simulink model "threePhase_SVPWM"  (R2022b)
settings: Solver=FixedStepAuto  StartTime=0.0  StopTime=0.02  RelTol=1e-3  EnableMultiTasking=on
values from neighbouring files (symbols this model uses):
  Vs = 230    [QuartusPath.m]
undefined symbols (not defined in the file or in its folder): Add, Shift
libraries: simulink x19, dspsrcs4 x3, dsphdlmathfun2 x1
settings Model: Creator=BAYINDIR  LastModifiedBy=BAYINDIR
settings OptimizationCC: BlockReduction=off  ConditionallyExecuteInputs=off
settings DebuggingCC: SingleTaskRateTransMsg=error

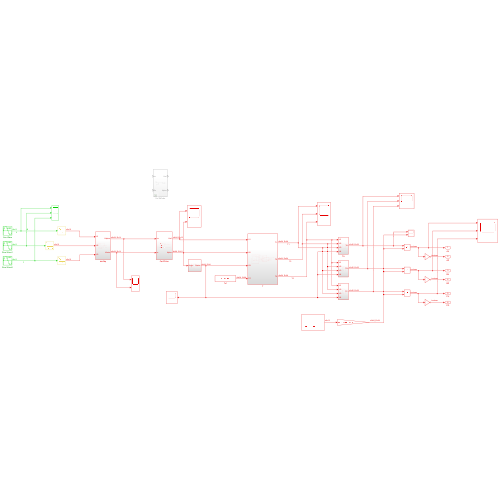
[thumbnail: Simulink's stored preview of the top-level diagram]
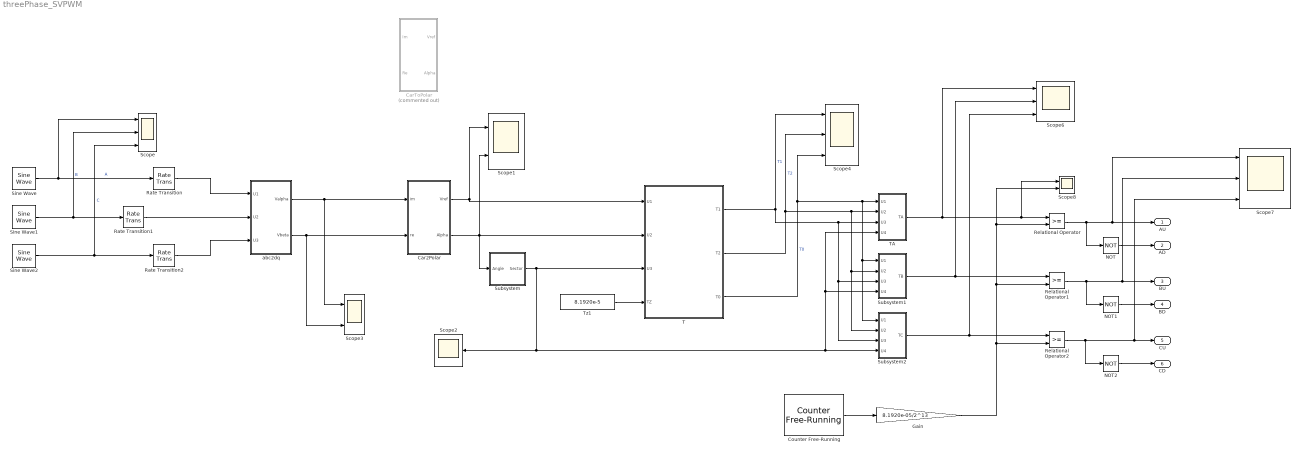
== system threePhase_SVPWM ==
  Car2Polar : Subsystem
  CarToPolar : Subsystem  Commented=on
  Counter Free-Running : simulink/Sources/Counter Free-Running  NumBits=13  tsamp=-1
  Gain : Gain  Gain=8.1920e-05/2^13  ParamDataTypeStr=fixdt(0,32,32)  OutDataTypeStr=fixdt(0,24,24)
  NOT : Logic  Operator=NOT  IconShape=distinctive  AllPortsSameDT=off  OutDataTypeStr=boolean
  NOT1 : Logic  Operator=NOT  IconShape=distinctive  AllPortsSameDT=off  OutDataTypeStr=boolean
  NOT2 : Logic  Operator=NOT  IconShape=distinctive  AllPortsSameDT=off  OutDataTypeStr=boolean
  Rate Transition : RateTransition  OutPortSampleTime=1/100000000
  Rate Transition1 : RateTransition  OutPortSampleTime=1/100000000
  Rate Transition2 : RateTransition  OutPortSampleTime=1/100000000
  Relational Operator : RelationalOperator  OutDataTypeStr=boolean  RndMeth=Simplest  InputSameDT=off
  Relational Operator1 : RelationalOperator  OutDataTypeStr=boolean  RndMeth=Simplest  InputSameDT=off
  Relational Operator2 : RelationalOperator  OutDataTypeStr=boolean  RndMeth=Simplest  InputSameDT=off
  Scope{,4,6..7} (4 alike) : Scope  NumInputPorts=3
  Scope1 : Scope  NumInputPorts=2
  Scope2 : Scope
  Scope3 : Scope  NumInputPorts=2
  Scope8 : Scope  NumInputPorts=2
  Sine Wave : dspsrcs4/Sine Wave  Amplitude=Vs  Frequency=50  Phase=0  SampleMode=Discrete  OutComplex=Real  CompMethod=Table lookup  TableSize=Speed  SampleTime=1/1000000  SamplesPerFrame=1  ResetState=Restart at time zero  OutputFrames=off  dataType=Fixed-point  wordLen=12  udDataType=sfix(16)  fracBitsMode=User-defined  numFracBits=0  OutDataTypeStr=fixdt(1,12,0)  LastOutDataTypeStr=fixdt(1,12,0)
  Sine Wave1 : dspsrcs4/Sine Wave  Amplitude=Vs  Frequency=50  Phase=2*pi/3  SampleMode=Discrete  OutComplex=Real  CompMethod=Table lookup  TableSize=Speed  SampleTime=1/1000000  SamplesPerFrame=1  ResetState=Restart at time zero  OutputFrames=off  dataType=Fixed-point  wordLen=12  udDataType=sfix(16)  fracBitsMode=User-defined  numFracBits=0  OutDataTypeStr=fixdt(1,12,0)  LastOutDataTypeStr=fixdt(1,12,0)
  Sine Wave2 : dspsrcs4/Sine Wave  Amplitude=Vs  Frequency=50  Phase=4*pi/3  SampleMode=Discrete  OutComplex=Real  CompMethod=Table lookup  TableSize=Speed  SampleTime=1/1000000  SamplesPerFrame=1  ResetState=Restart at time zero  OutputFrames=off  dataType=Fixed-point  wordLen=12  udDataType=sfix(16)  fracBitsMode=User-defined  numFracBits=0  OutDataTypeStr=fixdt(1,12,0)  LastOutDataTypeStr=fixdt(1,12,0)
  Subsystem : Subsystem
  Subsystem1 : Subsystem
  Subsystem2 : Subsystem
  T : Subsystem
  TA : Subsystem
  Tz1 : Constant  Value=8.1920e-5  OutDataTypeStr=fixdt(0,24,24)  SampleTime=-1
  abc2dq : Subsystem
  AU : Outport
  AD : Outport  Port=2
  BU : Outport  Port=3
  BD : Outport  Port=4
  CU : Outport  Port=5
  CD : Outport  Port=6
  wires:
  Sine Wave/1 -> Rate Transition/1, Scope/1  "A"
  Sine Wave1/1 -> Rate Transition1/1, Scope/2  "B"
  Sine Wave2/1 -> Rate Transition2/1, Scope/3  "C"
  Rate Transition/1 -> abc2dq/1(U1)
  Rate Transition1/1 -> abc2dq/2(U2)
  Rate Transition2/1 -> abc2dq/3(U3)
  Car2Polar/1(Vref) -> Scope1/1, T/1(U1)
  Car2Polar/2(Alpha) -> Scope1/2, Subsystem/1(Angle), T/2(U2)
  Subsystem/1(Sector) -> T/3(U3), TA/4(U4), Subsystem1/4(U4), Subsystem2/4(U4), Scope2/1
  Tz1/1 -> T/4(TZ)
  T/1(T1) -> TA/3(U3), Subsystem2/3(U3), Subsystem1/3(U3), Scope4/1  "T1"
  T/2(T2) -> Scope4/2, Subsystem1/2(U2), Subsystem2/2(U2), TA/2(U2)  "T2"
  T/3(T0) -> Scope4/3, Subsystem2/1(U1), Subsystem1/1(U1), TA/1(U1)  "T0"
  TA/1(TA) -> Scope8/1, Relational Operator/1, Scope6/1
  abc2dq/2(Vbeta) -> Car2Polar/2(re), Scope3/2
  abc2dq/1(Valpha) -> Scope3/1, Car2Polar/1(im)
  Subsystem1/1(TB) -> Relational Operator1/1, Scope6/2
  Subsystem2/1(TC) -> Relational Operator2/1, Scope6/3
  Counter Free-Running/1 -> Gain/1
  Relational Operator/1 -> NOT/1, Scope7/1, AU/1
  NOT/1 -> AD/1
  NOT1/1 -> BD/1
  Relational Operator1/1 -> NOT1/1, Scope7/2, BU/1
  Relational Operator2/1 -> Scope7/3, CU/1, NOT2/1
  NOT2/1 -> CD/1
  Gain/1 -> Scope8/2, Relational Operator/2, Relational Operator1/2, Relational Operator2/2

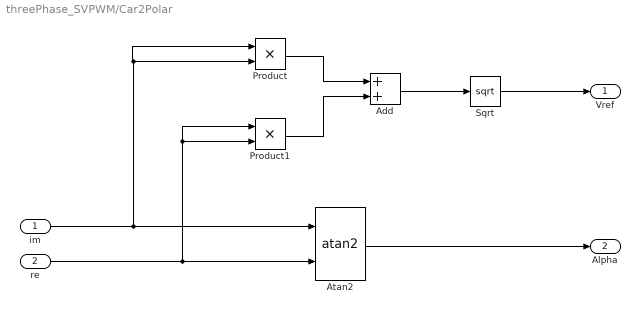
== system threePhase_SVPWM/Car2Polar ==
  im : Inport
  re : Inport  Port=2
  Add : Sum  OutDataTypeStr=fixdt(0,24,8)
  Atan2 : Trigonometry  Operator=atan2  ApproximationMethod=CORDIC  NumberOfIterations=13
  Product : Product  OutDataTypeStr=fixdt(1,48,28)
  Product1 : Product  OutDataTypeStr=fixdt(1,48,28)
  Sqrt : Sqrt  OutDataTypeStr=fixdt(0,24,12)
  Vref : Outport
  Alpha : Outport  Port=2
  wires:
  re/1 -> Product1/2, Product1/1, Atan2/2
  Atan2/1 -> Alpha/1
  im/1 -> Product/2, Product/1, Atan2/1
  Product/1 -> Add/1
  Product1/1 -> Add/2
  Add/1 -> Sqrt/1
  Sqrt/1 -> Vref/1

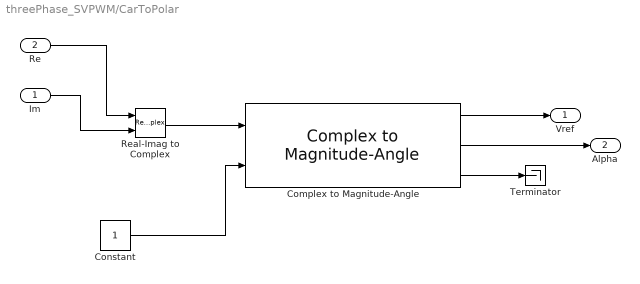
== system threePhase_SVPWM/CarToPolar ==
  Im : Inport
  Re : Inport  Port=2
  Complex to Magnitude-Angle : dsphdlmathfun2/Complex to Magnitude-Angle  NumIterationsSource=Property  NumIterations=12  OutputFormat=Magnitude and angle  AngleFormat=Radians  ScaleOutput=on  ScalingMethod=Shift-Add  SimulateUsing=Code generation
  Constant : Constant  OutDataTypeStr=boolean  SampleTime=-1
  Real-Imag to Complex : RealImagToComplex
  Terminator : Terminator
  Vref : Outport
  Alpha : Outport  Port=2
  wires:
  Im/1 -> Real-Imag to Complex/2
  Real-Imag to Complex/1 -> Complex to Magnitude-Angle/1
  Complex to Magnitude-Angle/3 -> Terminator/1
  Complex to Magnitude-Angle/2 -> Alpha/1
  Re/1 -> Real-Imag to Complex/1
  Constant/1 -> Complex to Magnitude-Angle/2
  Complex to Magnitude-Angle/1 -> Vref/1

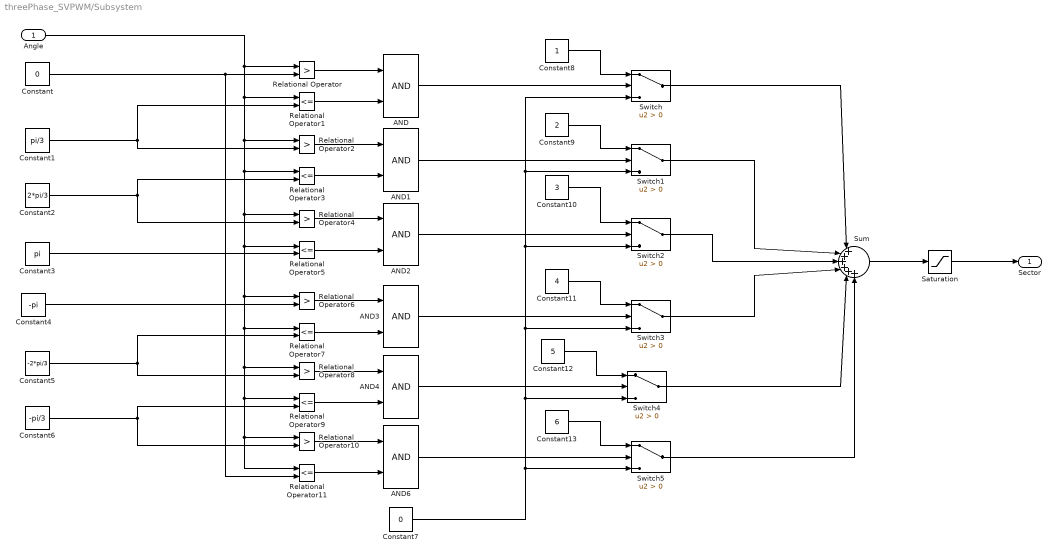
== system threePhase_SVPWM/Subsystem ==
  Angle : Inport
  AND{,1..4,6} (6 alike) : Logic  IconShape=distinctive  AllPortsSameDT=off  OutDataTypeStr=boolean
  Constant : Constant  Value=0  OutDataTypeStr=fixdt(1,27,24)  SampleTime=-1
  Constant1 : Constant  Value=pi/3  OutDataTypeStr=fixdt(1,27,24)  SampleTime=-1
  Constant10 : Constant  Value=3  OutDataTypeStr=fixdt(1,16,8)  SampleTime=-1
  Constant11 : Constant  Value=4  OutDataTypeStr=fixdt(1,16,8)  SampleTime=-1
  Constant12 : Constant  Value=5  OutDataTypeStr=fixdt(1,16,8)  SampleTime=-1
  Constant13 : Constant  Value=6  OutDataTypeStr=fixdt(1,16,8)  SampleTime=-1
  Constant2 : Constant  Value=2*pi/3  OutDataTypeStr=fixdt(1,27,24)  SampleTime=-1
  Constant3 : Constant  Value=pi  OutDataTypeStr=fixdt(1,27,24)  SampleTime=-1
  Constant4 : Constant  Value=-pi  OutDataTypeStr=fixdt(1,27,24)  SampleTime=-1
  Constant5 : Constant  Value=-2*pi/3  OutDataTypeStr=fixdt(1,27,24)  SampleTime=-1
  Constant6 : Constant  Value=-pi/3  OutDataTypeStr=fixdt(1,27,24)  SampleTime=-1
  Constant7 : Constant  Value=0  OutDataTypeStr=fixdt(1,16,8)  SampleTime=-1
  Constant8 : Constant  OutDataTypeStr=fixdt(1,16,8)  SampleTime=-1
  Constant9 : Constant  Value=2  OutDataTypeStr=fixdt(1,16,8)  SampleTime=-1
  Relational Operator{,2,4,6,8,10} (6 alike) : RelationalOperator  Operator=>  OutDataTypeStr=boolean  RndMeth=Simplest  InputSameDT=off
  Relational Operator{1,3,5,7,9,11} (6 alike) : RelationalOperator  Operator=<=  OutDataTypeStr=boolean  RndMeth=Simplest  InputSameDT=off
  Saturation : Saturate  UpperLimit=6  LowerLimit=1
  Sum : Sum  Inputs=|++++++  OutDataTypeStr=fixdt(0,16,8)
  Switch{,1..5} (6 alike) : Switch  Criteria=u2 > Threshold  SaturateOnIntegerOverflow=off  InputSameDT=off
  Sector : Outport
  wires:
  Angle/1 -> Relational Operator/1, Relational Operator10/1, Relational Operator11/1, Relational Operator9/1, Relational Operator8/1, Relational Operator7/1, Relational Operator6/1, Relational Operator5/1, Relational Operator4/1, Relational Operator3/1, Relational Operator2/1, Relational Operator1/1
  Relational Operator/1 -> AND/1
  AND4/1 -> Switch4/2
  Constant7/1 -> Switch5/3, Switch4/3, Switch3/3, Switch2/3, Switch1/3, Switch/3
  Saturation/1 -> Sector/1
  Constant9/1 -> Switch1/1
  Constant5/1 -> Relational Operator7/2, Relational Operator8/2
  Relational Operator6/1 -> AND3/1
  Constant1/1 -> Relational Operator2/2, Relational Operator1/2
  Switch1/1 -> Sum/2
  Relational Operator11/1 -> AND6/2
  Constant3/1 -> Relational Operator5/2
  Switch/1 -> Sum/1
  Sum/1 -> Saturation/1
  Constant10/1 -> Switch2/1
  Relational Operator5/1 -> AND2/2
  Constant13/1 -> Switch5/1
  Constant8/1 -> Switch/1
  Switch2/1 -> Sum/3
  AND1/1 -> Switch1/2
  AND6/1 -> Switch5/2
  Relational Operator10/1 -> AND6/1
  Switch5/1 -> Sum/6
  Constant2/1 -> Relational Operator4/2, Relational Operator3/2
  Relational Operator1/1 -> AND/2
  Constant4/1 -> Relational Operator6/2
  Relational Operator4/1 -> AND2/1
  Constant/1 -> Relational Operator11/2, Relational Operator/2
  Constant6/1 -> Relational Operator9/2, Relational Operator10/2
  Switch4/1 -> Sum/5
  Constant12/1 -> Switch4/1
  Constant11/1 -> Switch3/1
  Relational Operator7/1 -> AND3/2
  AND3/1 -> Switch3/2
  AND/1 -> Switch/2
  Switch3/1 -> Sum/4
  Relational Operator9/1 -> AND4/2
  Relational Operator3/1 -> AND1/2
  Relational Operator2/1 -> AND1/1
  AND2/1 -> Switch2/2
  Relational Operator8/1 -> AND4/1

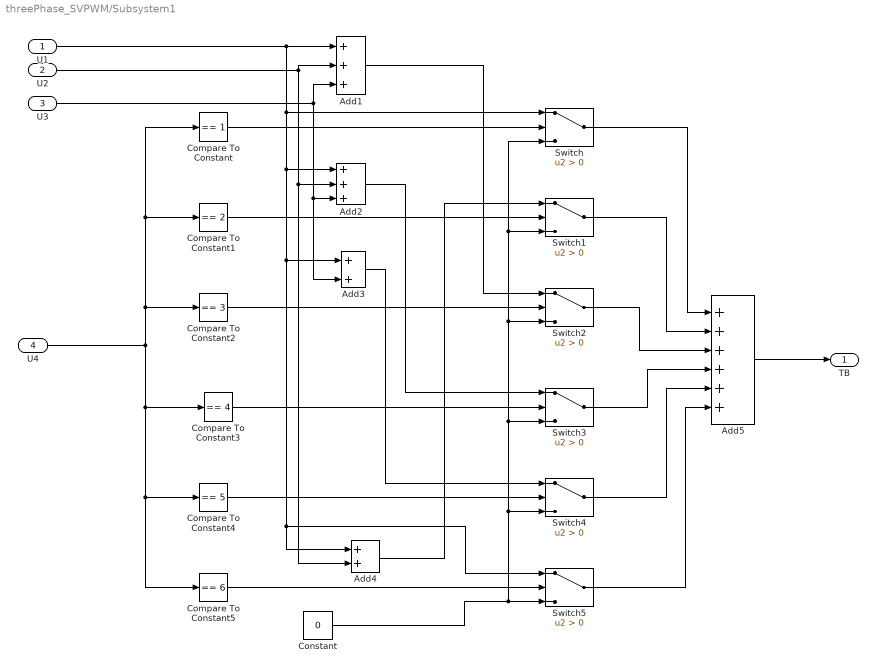
== system threePhase_SVPWM/Subsystem1 ==
  U1 : Inport
  U2 : Inport  Port=2
  U3 : Inport  Port=3
  U4 : Inport  Port=4
  Add1 : Sum  Inputs=+++  OutDataTypeStr=fixdt(0,24,24)
  Add2 : Sum  Inputs=+++  OutDataTypeStr=fixdt(0,24,24)
  Add3 : Sum  OutDataTypeStr=fixdt(0,24,24)
  Add4 : Sum  OutDataTypeStr=fixdt(0,24,24)
  Add5 : Sum  Inputs=++++++  OutDataTypeStr=fixdt(0,32,32)
  Compare To Constant : simulink/Logic and Bit Operations/Compare To Constant  relop===  const=1  OutDataTypeStr=boolean
  Compare To Constant1 : simulink/Logic and Bit Operations/Compare To Constant  relop===  const=2  OutDataTypeStr=boolean
  Compare To Constant2 : simulink/Logic and Bit Operations/Compare To Constant  relop===  const=3  OutDataTypeStr=boolean
  Compare To Constant3 : simulink/Logic and Bit Operations/Compare To Constant  relop===  const=4  OutDataTypeStr=boolean
  Compare To Constant4 : simulink/Logic and Bit Operations/Compare To Constant  relop===  const=5  OutDataTypeStr=boolean
  Compare To Constant5 : simulink/Logic and Bit Operations/Compare To Constant  relop===  const=6  OutDataTypeStr=boolean
  Constant : Constant  Value=0  OutDataTypeStr=uint8  SampleTime=-1
  Switch{,1..5} (6 alike) : Switch  Criteria=u2 > Threshold  OutDataTypeStr=fixdt(0,24,24)  SaturateOnIntegerOverflow=off  InputSameDT=off
  TB : Outport
  wires:
  U1/1 -> Switch5/1, Add4/1, Add3/1, Add2/1, Switch/1, Add1/1
  Compare To Constant4/1 -> Switch4/2
  Switch4/1 -> Add5/5
  Switch1/1 -> Add5/2
  U4/1 -> Compare To Constant2/1, Compare To Constant1/1, Compare To Constant/1, Compare To Constant4/1, Compare To Constant5/1, Compare To Constant3/1
  Compare To Constant1/1 -> Switch1/2
  Compare To Constant/1 -> Switch/2
  Constant/1 -> Switch4/3, Switch3/3, Switch2/3, Switch1/3, Switch/3, Switch5/3
  U2/1 -> Add2/2, Add4/2, Add1/2
  Compare To Constant5/1 -> Switch5/2
  Compare To Constant2/1 -> Switch2/2
  Switch5/1 -> Add5/6
  Switch/1 -> Add5/1
  Compare To Constant3/1 -> Switch3/2
  Switch2/1 -> Add5/3
  Switch3/1 -> Add5/4
  U3/1 -> Add1/3, Add2/3, Add3/2
  Add5/1 -> TB/1
  Add4/1 -> Switch1/1
  Add1/1 -> Switch2/1
  Add2/1 -> Switch3/1
  Add3/1 -> Switch4/1

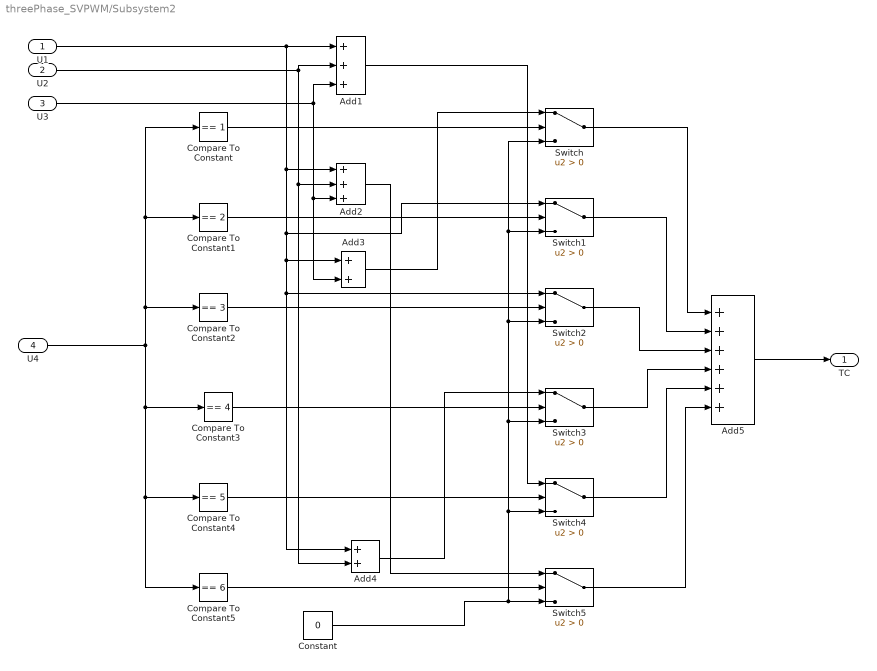
== system threePhase_SVPWM/Subsystem2 ==
  U1 : Inport
  U2 : Inport  Port=2
  U3 : Inport  Port=3
  U4 : Inport  Port=4
  Add1 : Sum  Inputs=+++  OutDataTypeStr=fixdt(0,24,24)
  Add2 : Sum  Inputs=+++  OutDataTypeStr=fixdt(0,24,24)
  Add3 : Sum  OutDataTypeStr=fixdt(0,24,24)
  Add4 : Sum  OutDataTypeStr=fixdt(0,24,24)
  Add5 : Sum  Inputs=++++++  OutDataTypeStr=fixdt(0,32,32)
  Compare To Constant : simulink/Logic and Bit Operations/Compare To Constant  relop===  const=1  OutDataTypeStr=boolean
  Compare To Constant1 : simulink/Logic and Bit Operations/Compare To Constant  relop===  const=2  OutDataTypeStr=boolean
  Compare To Constant2 : simulink/Logic and Bit Operations/Compare To Constant  relop===  const=3  OutDataTypeStr=boolean
  Compare To Constant3 : simulink/Logic and Bit Operations/Compare To Constant  relop===  const=4  OutDataTypeStr=boolean
  Compare To Constant4 : simulink/Logic and Bit Operations/Compare To Constant  relop===  const=5  OutDataTypeStr=boolean
  Compare To Constant5 : simulink/Logic and Bit Operations/Compare To Constant  relop===  const=6  OutDataTypeStr=boolean
  Constant : Constant  Value=0  OutDataTypeStr=uint8  SampleTime=-1
  Switch{,1..5} (6 alike) : Switch  Criteria=u2 > Threshold  OutDataTypeStr=fixdt(0,24,24)  SaturateOnIntegerOverflow=off  InputSameDT=off
  TC : Outport
  wires:
  U1/1 -> Add3/1, Add4/1, Switch2/1, Switch1/1, Add2/1, Add1/1
  Compare To Constant4/1 -> Switch4/2
  Switch4/1 -> Add5/5
  Switch1/1 -> Add5/2
  U4/1 -> Compare To Constant2/1, Compare To Constant1/1, Compare To Constant/1, Compare To Constant4/1, Compare To Constant5/1, Compare To Constant3/1
  Compare To Constant1/1 -> Switch1/2
  Compare To Constant/1 -> Switch/2
  Constant/1 -> Switch4/3, Switch3/3, Switch2/3, Switch1/3, Switch/3, Switch5/3
  U2/1 -> Add2/2, Add4/2, Add1/2
  Compare To Constant5/1 -> Switch5/2
  Compare To Constant2/1 -> Switch2/2
  Switch5/1 -> Add5/6
  Switch/1 -> Add5/1
  Compare To Constant3/1 -> Switch3/2
  Switch2/1 -> Add5/3
  Switch3/1 -> Add5/4
  U3/1 -> Add1/3, Add2/3, Add3/2
  Add5/1 -> TC/1
  Add3/1 -> Switch/1
  Add4/1 -> Switch3/1
  Add1/1 -> Switch4/1
  Add2/1 -> Switch5/1

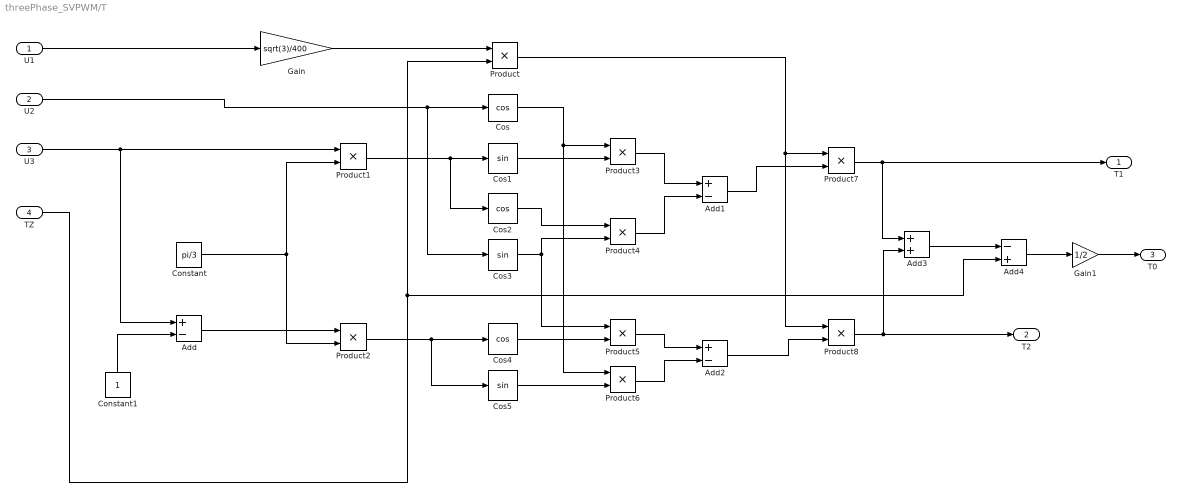
== system threePhase_SVPWM/T ==
  U1 : Inport
  U2 : Inport  Port=2
  U3 : Inport  Port=3
  TZ : Inport  Port=4
  Add : Sum  Inputs=+-  OutDataTypeStr=fixdt(1,16,8)
  Add1 : Sum  Inputs=+-
  Add2 : Sum  Inputs=+-
  Add3 : Sum  OutDataTypeStr=fixdt(0,24,24)
  Add4 : Sum  Inputs=-+  OutDataTypeStr=fixdt(0,24,24)
  Constant : Constant  Value=pi/3  OutDataTypeStr=fixdt(0,16,8)  SampleTime=-1
  Constant1 : Constant  OutDataTypeStr=fixdt(0,16,2)  SampleTime=-1
  Cos : Trigonometry  Operator=cos  ApproximationMethod=CORDIC  NumberOfIterations=13
  Cos1 : Trigonometry  ApproximationMethod=CORDIC  NumberOfIterations=13
  Cos2 : Trigonometry  Operator=cos  ApproximationMethod=CORDIC  NumberOfIterations=13
  Cos3 : Trigonometry  ApproximationMethod=CORDIC  NumberOfIterations=13
  Cos4 : Trigonometry  Operator=cos  ApproximationMethod=CORDIC  NumberOfIterations=13
  Cos5 : Trigonometry  ApproximationMethod=CORDIC  NumberOfIterations=13
  Gain : Gain  Gain=sqrt(3)/400  OutDataTypeStr=fixdt(0,12,10)
  Gain1 : Gain  Gain=1/2  OutDataTypeStr=fixdt(0,24,24)
  Product : Product  OutDataTypeStr=fixdt(0,20,18)
  Product{1..6} (6 alike) : Product  OutDataTypeStr=fixdt(1,16,8)
  Product7 : Product  OutDataTypeStr=fixdt(0,24,24)
  Product8 : Product  OutDataTypeStr=fixdt(1,24,24)
  T1 : Outport
  T2 : Outport  Port=2
  T0 : Outport  Port=3
  wires:
  Cos/1 -> Product6/1, Product3/1
  Product5/1 -> Add2/1
  Cos3/1 -> Product4/2, Product5/1
  Product/1 -> Product7/1, Product8/1
  Gain/1 -> Product/1
  Product2/1 -> Cos5/1, Cos4/1
  TZ/1 -> Product/2, Add4/2
  Constant/1 -> Product2/2, Product1/2
  Product8/1 -> T2/1, Add3/2
  Product1/1 -> Cos2/1, Cos1/1
  Constant1/1 -> Add/2
  Add/1 -> Product2/1
  Gain1/1 -> T0/1
  Cos5/1 -> Product6/2
  Add3/1 -> Add4/1
  Product3/1 -> Add1/1
  Cos1/1 -> Product3/2
  Product6/1 -> Add2/2
  Cos2/1 -> Product4/1
  Add2/1 -> Product8/2
  U1/1 -> Gain/1
  Add1/1 -> Product7/2
  Add4/1 -> Gain1/1
  Cos4/1 -> Product5/2
  Product4/1 -> Add1/2
  U3/1 -> Add/1, Product1/1
  U2/1 -> Cos3/1, Cos/1
  Product7/1 -> T1/1, Add3/1

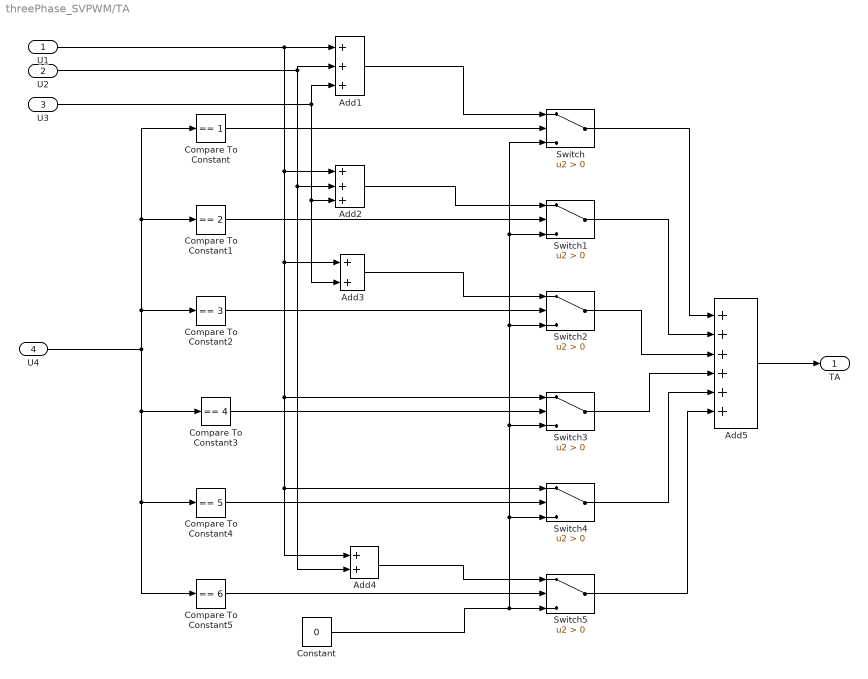
== system threePhase_SVPWM/TA ==
  U1 : Inport
  U2 : Inport  Port=2
  U3 : Inport  Port=3
  U4 : Inport  Port=4
  Add1 : Sum  Inputs=+++  OutDataTypeStr=fixdt(0,24,24)
  Add2 : Sum  Inputs=+++  OutDataTypeStr=fixdt(0,24,24)
  Add3 : Sum  OutDataTypeStr=fixdt(0,24,24)
  Add4 : Sum  OutDataTypeStr=fixdt(0,24,24)
  Add5 : Sum  Inputs=++++++  OutDataTypeStr=fixdt(0,32,32)
  Compare To Constant : simulink/Logic and Bit Operations/Compare To Constant  relop===  const=1  OutDataTypeStr=boolean
  Compare To Constant1 : simulink/Logic and Bit Operations/Compare To Constant  relop===  const=2  OutDataTypeStr=boolean
  Compare To Constant2 : simulink/Logic and Bit Operations/Compare To Constant  relop===  const=3  OutDataTypeStr=boolean
  Compare To Constant3 : simulink/Logic and Bit Operations/Compare To Constant  relop===  const=4  OutDataTypeStr=boolean
  Compare To Constant4 : simulink/Logic and Bit Operations/Compare To Constant  relop===  const=5  OutDataTypeStr=boolean
  Compare To Constant5 : simulink/Logic and Bit Operations/Compare To Constant  relop===  const=6  OutDataTypeStr=boolean
  Constant : Constant  Value=0  OutDataTypeStr=uint8  SampleTime=-1
  Switch{,1..5} (6 alike) : Switch  Criteria=u2 > Threshold  OutDataTypeStr=fixdt(0,24,24)  SaturateOnIntegerOverflow=off  InputSameDT=off
  TA : Outport
  wires:
  U1/1 -> Add3/1, Switch3/1, Switch4/1, Add4/1, Add2/1, Add1/1
  U2/1 -> Add2/2, Add4/2, Add1/2
  Add3/1 -> Switch2/1
  Add4/1 -> Switch5/1
  Compare To Constant/1 -> Switch/2
  Constant/1 -> Switch4/3, Switch3/3, Switch2/3, Switch1/3, Switch/3, Switch5/3
  Compare To Constant2/1 -> Switch2/2
  U4/1 -> Compare To Constant2/1, Compare To Constant1/1, Compare To Constant/1, Compare To Constant4/1, Compare To Constant5/1, Compare To Constant3/1
  Compare To Constant4/1 -> Switch4/2
  U3/1 -> Add1/3, Add2/3, Add3/2
  Add1/1 -> Switch/1
  Switch3/1 -> Add5/4
  Switch5/1 -> Add5/6
  Switch/1 -> Add5/1
  Switch1/1 -> Add5/2
  Compare To Constant5/1 -> Switch5/2
  Compare To Constant3/1 -> Switch3/2
  Switch4/1 -> Add5/5
  Add2/1 -> Switch1/1
  Compare To Constant1/1 -> Switch1/2
  Switch2/1 -> Add5/3
  Add5/1 -> TA/1

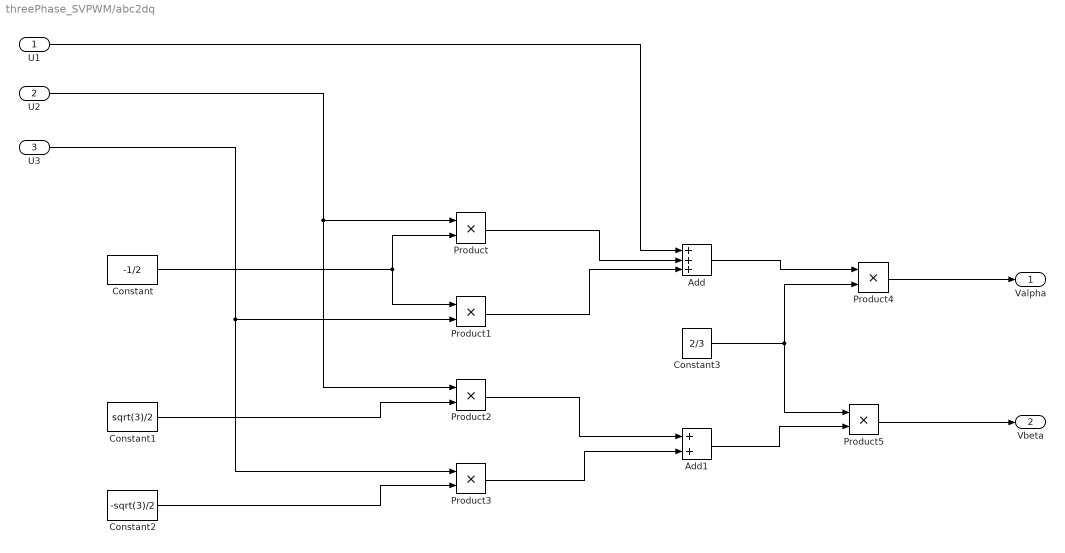
== system threePhase_SVPWM/abc2dq ==
  U1 : Inport
  U2 : Inport  Port=2
  U3 : Inport  Port=3
  Add : Sum  Inputs=+++  OutDataTypeStr=fixdt(1,12,2)
  Add1 : Sum  OutDataTypeStr=fixdt(1,12,2)
  Constant : Constant  Value=-1/2  OutDataTypeStr=fixdt(1,10,8)  SampleTime=-1
  Constant1 : Constant  Value=sqrt(3)/2  OutDataTypeStr=fixdt(0,10,8)  SampleTime=-1
  Constant2 : Constant  Value=-sqrt(3)/2  OutDataTypeStr=fixdt(1,10,8)  SampleTime=-1
  Constant3 : Constant  Value=2/3  OutDataTypeStr=fixdt(0,10,8)  SampleTime=-1
  Product : Product  OutDataTypeStr=fixdt(1,12,4)
  Product1 : Product  OutDataTypeStr=fixdt(1,12,4)
  Product2 : Product  OutDataTypeStr=fixdt(1,12,2)
  Product3 : Product  OutDataTypeStr=fixdt(1,12,2)
  Product4 : Product  OutDataTypeStr=fixdt(1,24,14)
  Product5 : Product  OutDataTypeStr=fixdt(1,24,14)
  Valpha : Outport
  Vbeta : Outport  Port=2
  wires:
  Add1/1 -> Product5/2
  Constant3/1 -> Product5/1, Product4/2
  Constant/1 -> Product/2, Product1/1
  Constant2/1 -> Product3/2
  Product/1 -> Add/2
  Constant1/1 -> Product2/2
  Product3/1 -> Add1/2
  Add/1 -> Product4/1
  U1/1 -> Add/1
  Product1/1 -> Add/3
  U3/1 -> Product3/1, Product1/2
  U2/1 -> Product2/1, Product/1
  Product2/1 -> Add1/1
  Product5/1 -> Vbeta/1
  Product4/1 -> Valpha/1
